simulink model "m_k_m_system"  (R2019b)
settings: Solver=VariableStepAuto  StartTime=0.0  StopTime=10  FixedStep=1e-3  RelTol=1e-5  AbsTol=1e-5
libraries: simulink x1
settings Model: OrderedModelArguments=off  Creator=19398  LastModifiedBy=19398

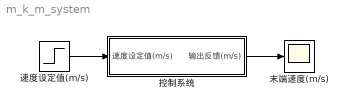
== system m_k_m_system ==
  控制系统 : Subsystem
  末端速度(m/s) : Scope
  速度设定值(m/s) : Step  Time=2  After=10  SampleTime=0
  wires:
  速度设定值(m/s)/1 -> 控制系统/1(速度设定值(m/s))
  控制系统/1(输出反馈(m/s)) -> 末端速度(m/s)/1

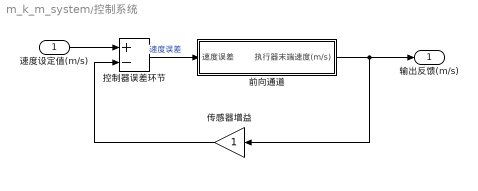
== system m_k_m_system/控制系统 ==
  速度设定值(m/s) : Inport
  传感器增益 : Gain
  前向通道 : Subsystem
  控制器误差环节 : Sum  Inputs=+-
  输出反馈(m/s) : Outport
  wires:
  速度设定值(m/s)/1 -> 控制器误差环节/1
  传感器增益/1 -> 控制器误差环节/2
  控制器误差环节/1 -> 前向通道/1(速度误差)  "速度误差"
  前向通道/1(执行器末端速度(m/s)) -> 输出反馈(m/s)/1, 传感器增益/1

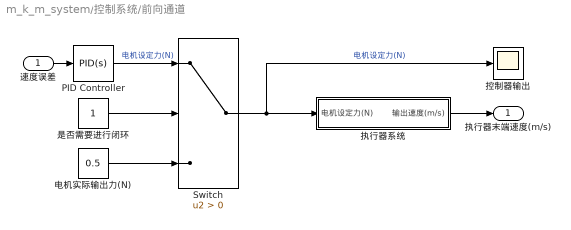
== system m_k_m_system/控制系统/前向通道 ==
  速度误差 : Inport
  PID Controller : simulink/Continuous/PID Controller  Controller=PID  Form=Parallel  TimeDomain=Continuous-time  SampleTime=-1  IntegratorMethod=Forward Euler  FilterMethod=Forward Euler  ControllerParametersSource=internal  P=1.20757381305832  I=9.42190600466165  D=0.0229368818155682  UseFilter=on  N=1091.39224421761  TunerSelectOption=Transfer Function Based (PID Tuner App)  InitialConditionSource=internal  InitialConditionForIntegrator=0  InitialConditionForFilter=0  DifferentiatorICPrevScaledInput=0  ExternalReset=none  TrackingMode=off  Kt=1  LimitOutput=off  UpperSaturationLimit=inf  LowerSaturationLimit=-inf  LinearizeAsGain=on  AntiWindupMode=none  Kb=1  POutMin=[]  POutMax=[]  IOutMin=[-10]  IOutMax=[10]  DOutMin=[]  DOutMax=[]  NOutMin=[]  NOutMax=[]  SumOutMin=[]  SumOutMax=[]  SaturationOutMin=[]  SaturationOutMax=[]  PParamMin=[]  PParamMax=[]  IParamMin=[]  IParamMax=[]  DParamMin=[]  DParamMax=[]  NParamMin=[]  NParamMax=[]  KbParamMin=[]  KbParamMax=[]  KtParamMin=[]  KtParamMax=[]  KbOutMin=[]  KbOutMax=[]  KtOutMin=[]  KtOutMax=[]  IntegratorOutMin=[]  IntegratorOutMax=[]  FilterOutMin=[]  FilterOutMax=[]  SumI1OutMin=[]  SumI1OutMax=[]  SumI2OutMin=[]  SumI2OutMax=[]  SumI3OutMin=[]  SumI3OutMax=[]  SumI4OutMin=[]  SumI4OutMax=[]  SumDOutMin=[]  SumDOutMax=[]  DifferentiatorOutMin=[]  DifferentiatorOutMax=[]  FilterDiffOutCoefMin=[]  FilterDiffOutCoefMax=[]  ReciprocalOutMin=[]  ReciprocalOutMax=[]  SumDenOutMin=[]  SumDenOutMax=[]  SumNumOutMin=[]  SumNumOutMax=[]  DivideOutMin=[]  DivideOutMax=[]  IntegratorContinuousStateAttributes=''  IntegratorStateMustResolveToSignalObject=off  IntegratorRTWStateStorageClass=Auto  FilterContinuousStateAttributes=''  FilterStateMustResolveToSignalObject=off  FilterRTWStateStorageClass=Auto  ParallelPVariant=InternalParameters  IdealPVariant=Disabled  IVariant=InternalParameters  DVariant=InternalParameters  IntegratorVariant=Continuous  SatVariant=Disabled  AWVariant=Passthrough  PCopyVariant=Disabled  TRVariant=Disabled  FdbkBlocksVariant=Forward  IdealPFdbkVariant=Disabled  SatFdbkVariant=Disabled  DerivativeFilterVariant=ContFilter  NVariant=InternalParameters  NCopyVariant=Disabled  FilterICVariant=InternalICsFilter  IntegratorICVariant=InternalICs  ExternalResetVariant=Disabled  TRSumVariant=Passthrough  SumFdbkVariant=Disabled  SumVariant=Sum_PID
  Switch : Switch  Criteria=u2 > Threshold
  执行器系统 : Subsystem  mask{IfResilient=1}
      mask prompts: IfResilient "系统是否具有弹性"
  控制器输出 : Scope
  是否需要进行闭环 : Constant
  电机实际输出力(N) : Constant  Value=0.5
  执行器末端速度(m/s) : Outport
  wires:
  速度误差/1 -> PID Controller/1
  执行器系统/1(输出速度(m/s)) -> 执行器末端速度(m/s)/1
  Switch/1 -> 控制器输出/1, 执行器系统/1(电机设定力(N))  "电机设定力(N)"
  是否需要进行闭环/1 -> Switch/2
  PID Controller/1 -> Switch/1  "电机设定力(N)"
  电机实际输出力(N)/1 -> Switch/3

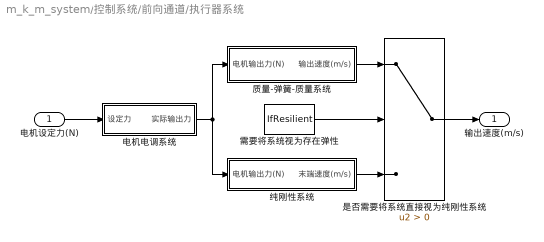
== system m_k_m_system/控制系统/前向通道/执行器系统 ==
  电机设定力(N) : Inport
  是否需要将系统直接视为纯刚性系统 : Switch  Criteria=u2 > Threshold
  电机电调系统 : Subsystem  mask{Fre=800, MaxForce=20}
      mask prompts: Fre "系统的截止频率(Hz)"; MaxForce "电机输出最大的力(N)"
  纯刚性系统 : Subsystem  mask{TotalMass=0.15, niu=0.05}
      mask prompts: TotalMass "总质量"; niu "动摩擦因数"
  质量-弹簧-质量系统 : Subsystem  mask{InitialLenOfSpring=1, k=100, m1=0.1, m2=0.05, niu=0.05}
      mask prompts: InitialLenOfSpring "弹簧原始长度(m)"; k "弹簧劲度系数(N/m)"; m1 "直接受力物体质量(kg)"; m2 "速度被控物体质量(kg)"; niu "地面的动摩擦因数"
  需要将系统视为存在弹性 : Constant  Value=IfResilient
  输出速度(m/s) : Outport
  wires:
  电机设定力(N)/1 -> 电机电调系统/1(设定力)
  电机电调系统/1(实际输出力) -> 质量-弹簧-质量系统/1(电机输出力(N)), 纯刚性系统/1(电机输出力(N))
  质量-弹簧-质量系统/1(输出速度(m/s)) -> 是否需要将系统直接视为纯刚性系统/1
  纯刚性系统/1(末端速度(m/s)) -> 是否需要将系统直接视为纯刚性系统/3
  是否需要将系统直接视为纯刚性系统/1 -> 输出速度(m/s)/1
  需要将系统视为存在弹性/1 -> 是否需要将系统直接视为纯刚性系统/2

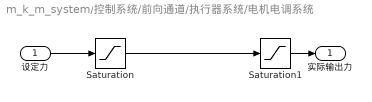
== system m_k_m_system/控制系统/前向通道/执行器系统/电机电调系统 ==
  设定力 : Inport
  Saturation : Saturate  UpperLimit=MaxForce  LowerLimit=-MaxForce
  Saturation1 : Saturate  UpperLimit=MaxForce  LowerLimit=-MaxForce
  实际输出力 : Outport
  wires:
  设定力/1 -> Saturation/1
  Saturation/1 -> Saturation1/1
  Saturation1/1 -> 实际输出力/1

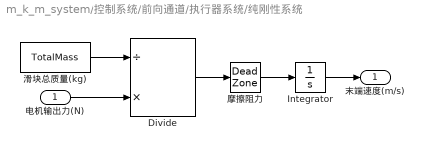
== system m_k_m_system/控制系统/前向通道/执行器系统/纯刚性系统 ==
  电机输出力(N) : Inport
  Divide : Product  Inputs=/*
  Integrator : Integrator
  摩擦阻力 : DeadZone  LowerValue=-niu  UpperValue=niu  SaturateOnIntegerOverflow=on
  滑块总质量(kg) : Constant  Value=TotalMass
  末端速度(m/s) : Outport
  wires:
  滑块总质量(kg)/1 -> Divide/1
  电机输出力(N)/1 -> Divide/2
  Divide/1 -> 摩擦阻力/1
  Integrator/1 -> 末端速度(m/s)/1
  摩擦阻力/1 -> Integrator/1

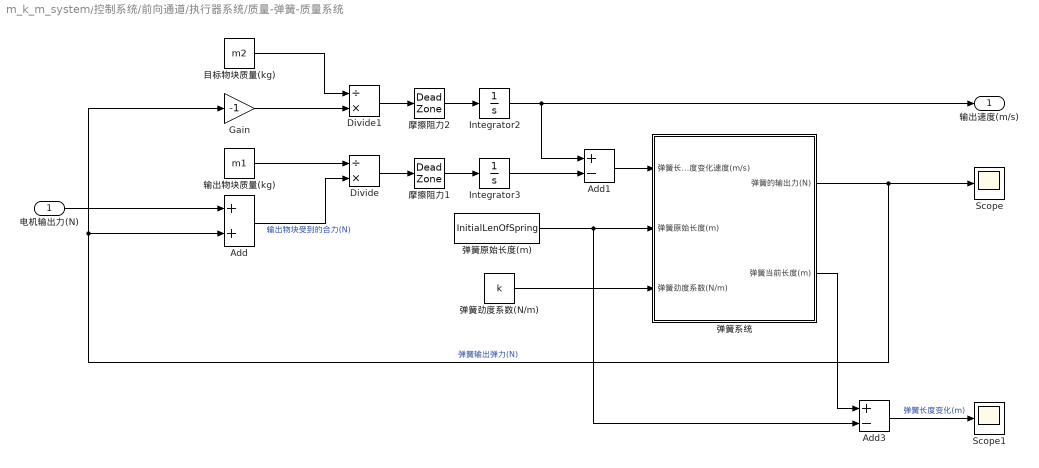
== system m_k_m_system/控制系统/前向通道/执行器系统/质量-弹簧-质量系统 ==
  电机输出力(N) : Inport
  Add : Sum
  Add1 : Sum  Inputs=+-
  Add3 : Sum  Inputs=+-
  Divide : Product  Inputs=/*
  Divide1 : Product  Inputs=/*
  Gain : Gain  Gain=-1
  Integrator2 : Integrator
  Integrator3 : Integrator
  Scope : Scope
  Scope1 : Scope
  弹簧劲度系数(N/m) : Constant  Value=k
  弹簧原始长度(m) : Constant  Value=InitialLenOfSpring
  弹簧系统 : Subsystem
  摩擦阻力1 : DeadZone  LowerValue=0  UpperValue=0  SaturateOnIntegerOverflow=on
  摩擦阻力2 : DeadZone  LowerValue=0  UpperValue=0  SaturateOnIntegerOverflow=on
  目标物块质量(kg) : Constant  Value=m2
  输出物块质量(kg) : Constant  Value=m1
  输出速度(m/s) : Outport
  wires:
  弹簧原始长度(m)/1 -> 弹簧系统/2(弹簧原始长度(m)), Add3/2
  弹簧系统/1(弹簧的输出力(N)) -> Gain/1, Add/2, Scope/1  "弹簧输出弹力(N)"
  目标物块质量(kg)/1 -> Divide1/1
  弹簧劲度系数(N/m)/1 -> 弹簧系统/3(弹簧劲度系数(N/m))
  输出物块质量(kg)/1 -> Divide/1
  Divide1/1 -> 摩擦阻力2/1
  Divide/1 -> 摩擦阻力1/1
  Add/1 -> Divide/2  "输出物块受到的合力(N)"
  Gain/1 -> Divide1/2
  Add3/1 -> Scope1/1  "弹簧长度变化(m)"
  电机输出力(N)/1 -> Add/1
  Add1/1 -> 弹簧系统/1(弹簧长度变化速度(m/s))
  摩擦阻力2/1 -> Integrator2/1
  摩擦阻力1/1 -> Integrator3/1
  Integrator2/1 -> 输出速度(m/s)/1, Add1/1
  Integrator3/1 -> Add1/2
  弹簧系统/2(弹簧当前长度(m)) -> Add3/1

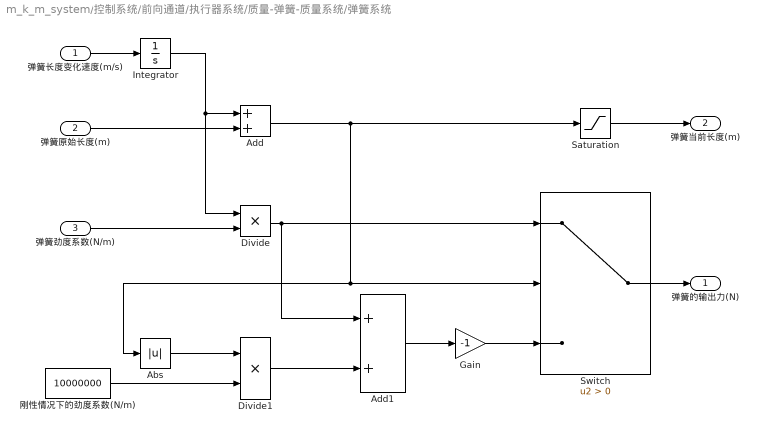
== system m_k_m_system/控制系统/前向通道/执行器系统/质量-弹簧-质量系统/弹簧系统 ==
  弹簧长度变化速度(m/s) : Inport
  弹簧原始长度(m) : Inport  Port=2
  弹簧劲度系数(N/m) : Inport  Port=3
  Abs : Abs
  Add : Sum
  Add1 : Sum
  Divide : Product  Inputs=**
  Divide1 : Product  Inputs=**
  Gain : Gain  Gain=-1
  Integrator : Integrator
  Saturation : Saturate  UpperLimit=10000000000  LowerLimit=0
  Switch : Switch  Criteria=u2 > Threshold
  刚性情况下的劲度系数(N/m) : Constant  Value=10000000
  弹簧的输出力(N) : Outport
  弹簧当前长度(m) : Outport  Port=2
  wires:
  弹簧长度变化速度(m/s)/1 -> Integrator/1
  Integrator/1 -> Divide/1, Add/1
  弹簧原始长度(m)/1 -> Add/2
  Add/1 -> Switch/2, Abs/1, Saturation/1
  Saturation/1 -> 弹簧当前长度(m)/1
  Switch/1 -> 弹簧的输出力(N)/1
  Divide/1 -> Add1/1, Switch/1
  弹簧劲度系数(N/m)/1 -> Divide/2
  Add1/1 -> Gain/1
  Abs/1 -> Divide1/1
  Divide1/1 -> Add1/2
  刚性情况下的劲度系数(N/m)/1 -> Divide1/2
  Gain/1 -> Switch/3
